simulink model "task4_simulink"  (R2024b)
settings: Solver=ode45  StartTime=0.0  StopTime=100  RelTol=1e-6  AbsTol=1e-8
undefined symbols (not defined in the file): delta_trim, params, T_trim, x_trim
libraries: aerolibatmos2 x1
settings Model: Creator=Admin  LastModifiedBy=david

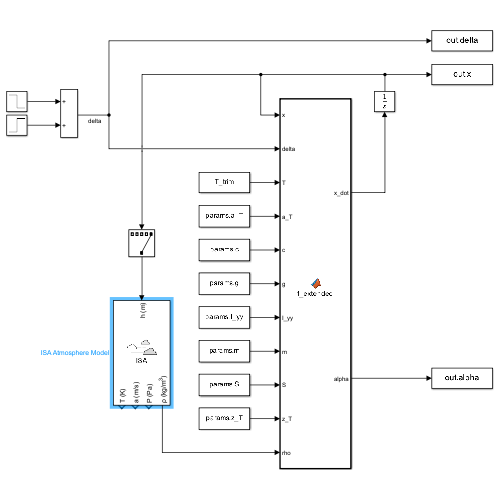
[thumbnail: Simulink's stored preview of the top-level diagram]
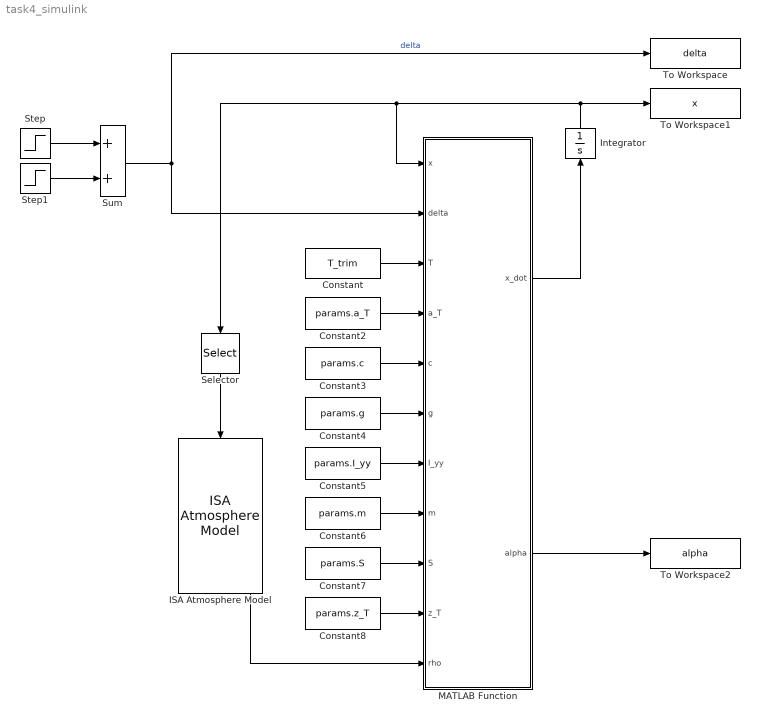
== system task4_simulink ==
  Constant : Constant  Value=T_trim
  Constant2 : Constant  Value=params.a_T
  Constant3 : Constant  Value=params.c
  Constant4 : Constant  Value=params.g
  Constant5 : Constant  Value=params.I_yy
  Constant6 : Constant  Value=params.m
  Constant7 : Constant  Value=params.S
  Constant8 : Constant  Value=params.z_T
  ISA Atmosphere Model : aerolibatmos2/ISA Atmosphere Model  useExtended=off  action=Warning  custom=off  viscosityOut=off  g=9.80665  gamma=1.4  R=287.0531  L=0.0065  h_trop=11000  h_strat=20000  rho0=1.225  P0=101325  T0=288.15  h0=0  S=110.4  Tref=273.15  muref=1.716e-5
  Integrator : Integrator  InitialCondition=x_trim
  MATLAB Function : MATLAB Function  TreatAsAtomicUnit=on
  Selector : Selector  InputPortWidth=5  IndexOptions=Index vector (dialog)  Indices=[5]  OutputSizes=1
  Step : Step  Time=5  Before=delta_trim  After=delta_trim - pi/180  SampleTime=0
  Step1 : Step  Time=10  After=(pi/180)  SampleTime=0
  Sum : Sum
  To Workspace : ToWorkspace  VariableName=delta  SampleTime=-1
  To Workspace1 : ToWorkspace  VariableName=x  SaveFormat=Structure  SampleTime=-1
      settings: Save2DSignal=2-D array (concatenate along first dimension)
  To Workspace2 : ToWorkspace  VariableName=alpha  SaveFormat=Timeseries  SampleTime=-1
  wires:
  Step1/1 -> Sum/2
  Step/1 -> Sum/1
  Sum/1 -> MATLAB Function/2(delta), To Workspace/1  "delta"
  MATLAB Function/1(x_dot) -> Integrator/1
  Integrator/1 -> MATLAB Function/1(x), Selector/1, To Workspace1/1
  Constant/1 -> MATLAB Function/3(T)
  Constant2/1 -> MATLAB Function/4(a_T)
  Constant3/1 -> MATLAB Function/5(c)
  Constant4/1 -> MATLAB Function/6(g)
  Constant5/1 -> MATLAB Function/7(I_yy)
  Constant6/1 -> MATLAB Function/8(m)
  Constant7/1 -> MATLAB Function/9(S)
  Constant8/1 -> MATLAB Function/10(z_T)
  MATLAB Function/2(alpha) -> To Workspace2/1
  ISA Atmosphere Model/4 -> MATLAB Function/11(rho)
  Selector/1 -> ISA Atmosphere Model/1

== matlab function task4_simulink/MATLAB Function ==
  data: x input; delta input; T input; a_T input; c input; g input; I_yy input; m input; S input; z_T input; x_dot output; alpha output; rho input
function [x_dot, alpha] = f_extended(x, delta, T, a_T, c, g, I_yy, m, S, z_T, rho)
        u = x(1);
        w = x(2);
        q = x(3);
        theta = x(4);
        % h = x(5);

        if (u ~= 0)
            alpha = atan(w / u);
        else
            alpha = 0;
        end

        V = sqrt(u ^ 2 + w ^ 2);

        c_L0 = 0.895;
        c_L_alpha = 5.01;
        c_L_delta = 0.722;
        c_D0 = 0.177;
        c_D_alpha = 0.232;
        c_D_alpha2 = 1.393;
        c_M0 = -0.046;
        c_M_alpha = -1.087;
        c_M_q = -7.055;
        c_M_delta = -1.88;

        c_L = @(alpha, delta) c_L0 + c_L_alpha * alpha + c_L_delta * delta;
        c_D = @(alpha) c_D0 + c_D_alpha * alpha + c_D_alpha2 * alpha ^ 2;
        c_M = @(alpha, delta, V, q) c_M0 + c_M_alpha * alpha + c_M_q * (c / V) * q + c_M_delta * delta;

        c_L = c_L(alpha, delta);
        c_D = c_D(alpha);
        c_M = c_M(alpha, delta, V, q);

        L = 0.5 * rho * V ^ 2 * S * c_L;
        D = 0.5 * rho * V ^ 2 * S * c_D;

        X_A = L * sin(alpha) - D * cos(alpha);
        Z_A = -L * cos(alpha) - D * sin(alpha);
        M_A = 0.5 * rho * V ^ 2 * S * c * c_M;

        X_T = T * cos(a_T);
        Z_T = -T * sin(a_T);
        M_T = T * z_T;

        u_dot = -q * w - g * sin(theta) + 1 / m * X_A + 1 / m * X_T;
        w_dot = q * u + g * cos(theta) + 1 / m * Z_A + 1 / m * Z_T;
        q_dot = 1 / I_yy * M_A + 1 / I_yy * M_T;
        theta_dot = q;
        h_dot = u * sin(theta) - w * cos(theta);

        x_dot = [u_dot; w_dot; q_dot; theta_dot; h_dot];
    end
